simulink library "libMdl_Imm"  (R2019b)
settings: Solver=VariableStepAuto  StartTime=0.0  StopTime=10.0  RelTol=1e-3
undefined symbols (not defined in the file or in its folder): imm_measurement_fcns, imm_mu_sample_time, imm_residuum_fcns, imm_sample_time, imm_state_transition_fcns, mu_0, P_0_imm, Pi, x_0_imm
settings Model: Creator=hwinter  LastModifiedBy=Hanno
settings DataIOCC: ReturnWorkspaceOutputs=off
settings DebuggingCC: ArithmeticOperatorsInVariantConditions=warning
settings SFSimCC: SimUseLocalCustomCode=off  CustomCodeUndefinedFunction=UseInterfaceOnly
settings RTWCC: RTWUseLocalCustomCode=off

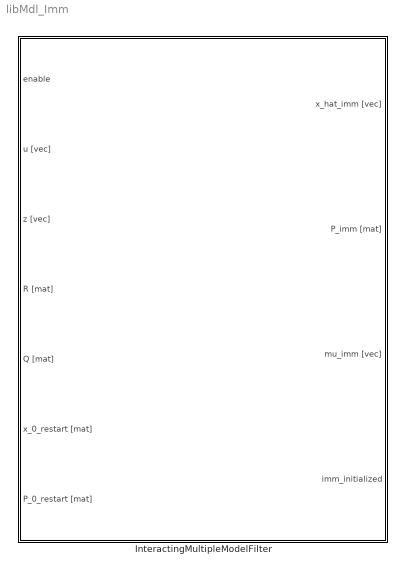
== system libMdl_Imm ==
  InteractingMultipleModelFilter : Subsystem  SystemSampleTime=mv_sample_time  mask(Interacting Multiple Model Filter){mv_sample_time=imm_sample_time, mv_mu_sample_time=imm_mu_sample_time, mv_x_0=x_0_imm, mv_P_0=P_0_imm, mv_pi=Pi, mv_mu_0=mu_0, mv_state_transition_functions=imm_state_transition_fcns, mv_measurement_functions=imm_measurement_fcns, mv_residuum_functions=imm_residuum_fcns}
      mask prompts: mv_sample_time "Sample Time:"; mv_mu_sample_time "Model Likelihood Sample Time:"; mv_x_0 "Initial State:"; mv_P_0 "Initial Covariance:"; mv_pi "Pi:"; mv_mu_0 "mu_0:"; mv_state_transition_functions "State Transition Functions:"; mv_measurement_functions "Measurement Functions:"; mv_residuum_functions "Residuum Functions:"
      mask help:
      | Sample Time:
      | Sample time of the block in seconds
      |
      | Initial State:
      | Initial state in correspondens to the state transition functions
      |
      | Initial Covariance:
      | Initial covariance matrix corresponding to the initial state, defined previously
      |
      | Pi:
      | Model Transition probability matrix
      |
      | mu_0:
      | Initial model probabilities
      |
      | State Transition Functions:
      | Names of the state transition functions, which have to be defined somewhere in the Matlab workspace
      | (example: {stateTransitionFcn1,stateTransitionFcn2})
      |
      | Measurement Functions:
      | Names of the measurement functions, which have to be defined somewhere in the Matlab workspace
      | (example: {measurementFcn1,measurementFcn2})
      |
      | Residuum Functions:
      | Optional functions to calculate measurement innovation (e.g. if angles are included). Leave '[]' if not needed.
      | (example: {residuumFcn1,residuumFcnFcn2})
      mask init:
      | % [mv_state_transition_functions,mv_measurement_functions] = simFcn_Imm_MaskInit(mv_state_transition_functions,mv_measurement_functions);
      | [mv_state_transition_functions,mv_measurement_functions,mv_residuum_functions] = simFcn_Imm_MaskInit(mv_state_transition_functions,mv_measurement_functions,mv_residuum_functions);
      mask Display:
      | str1 = sprintf('\\color{black}{\\bfIMM Filter}\n\n');
      | str2 = sprintf('Sample Time: %0.2f\n',mv_sample_time);
      | str3 = sprintf('Model Likelihood Sample Time: %0.2f\n\n',mv_mu_sample_time);
      | if length(mv_x_0) <= 3
      |     str4 = sprintf('x_0: %s\n',mat2str(mv_x_0,5));
      | else
      |     str4 = sprintf('x_0: [...]\n');
      | end % if
      | if length(mv_P_0) == 1
      |     str5 = sprintf('P_0: %0.2f\n\n',mv_P_0);
      | else
      |     str5 = sprintf('P_0: [...]\n\n');
      | end % if
      | str6 = sprintf('\\Pi: [...]\n');
      | if length(mv_mu_0) <= 3
      |     str7 = sprintf('\\mu_0: %s\n\n',mat2str(mv_mu_0,5));
      | else
      |     str7 = sprintf('\\mu_0: [...]\n\n');
      | end % if
      | str8 = sprintf('State Transition Functions: [...]\n');
      | str9 = sprintf('Measurement Functions: [...]\n');
      | if isempty(mv_residuum_functions)
      |     str10 = '';
      | else
      |     str10 = sprintf('Residuum Functions: [...]');
      | end % if
      | 
      | str = [str1,str2,str3,str4,str5,str6,str7,str8,str9,str10];
      | 
      | text( 0.5,0.5, ...
      |       str, ...
      |       'horizontalAlignment', 'center', ...
      |       'texmode','on' ...
      |     )

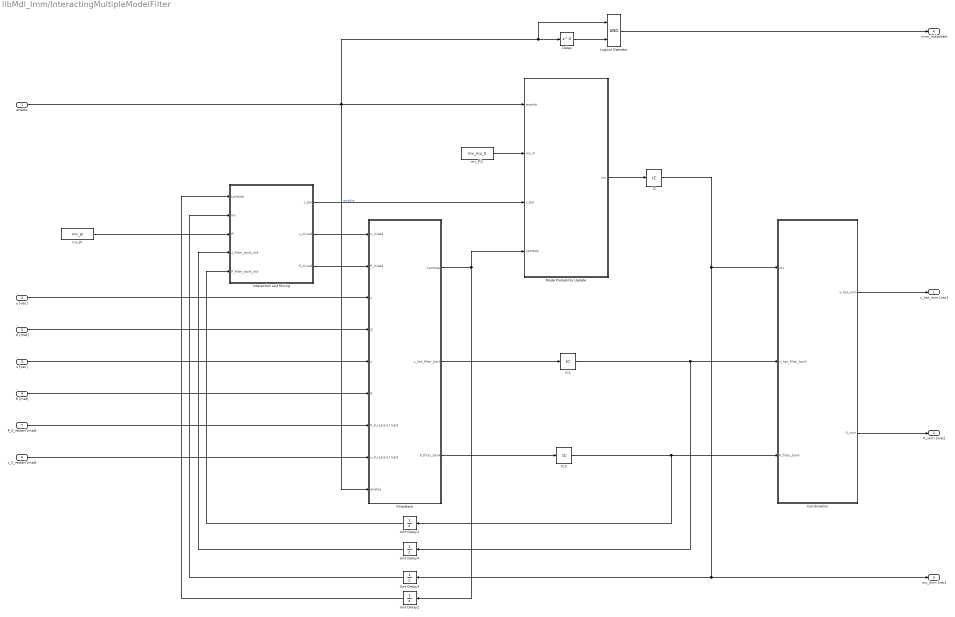
== system libMdl_Imm/InteractingMultipleModelFilter ==
  enable : Inport  SampleTime=mv_sample_time
  u [vec] : Inport  Port=2  SampleTime=mv_sample_time
  z [vec] : Inport  Port=3  SampleTime=mv_sample_time
  R [mat] : Inport  Port=4  SampleTime=mv_sample_time
  Q [mat] : Inport  Port=5  SampleTime=mv_sample_time
  x_0_restart [mat] : Inport  Port=6  SampleTime=mv_sample_time
  P_0_restart [mat] : Inport  Port=7  SampleTime=mv_sample_time
  Combination : Subsystem
  Delay : Delay
  FilterBank : Subsystem  SystemSampleTime=mv_sample_time
  IC : InitialCondition  Value=mv_mu_0
  IC1 : InitialCondition  Value=mv_x_0
  IC2 : InitialCondition  Value=mv_P_0
  Interaction and Mixing : Subsystem  TreatAsAtomicUnit=on
  Logical Operator : Logic  AllPortsSameDT=off  OutDataTypeStr=boolean
  Mode Probability Update : Subsystem
  Unit Delay1 : UnitDelay  InitialCondition=mv_P_0  SampleTime=-1  HasFrameUpgradeWarning=on
  Unit Delay2 : UnitDelay  InitialCondition=NaN(size(mv_mu_0))  SampleTime=-1  HasFrameUpgradeWarning=on
  Unit Delay3 : UnitDelay  InitialCondition=mv_mu_0  SampleTime=-1  HasFrameUpgradeWarning=on
  Unit Delay4 : UnitDelay  InitialCondition=mv_x_0  SampleTime=-1  HasFrameUpgradeWarning=on
  mv_Pi : Constant  Value=mv_pi
  mv_Pi1 : Constant  Value=mv_mu_0
  x_hat_imm [vec] : Outport  VectorParamsAs1DForOutWhenUnconnected=off
  P_imm [mat] : Outport  Port=2  VectorParamsAs1DForOutWhenUnconnected=off
  mu_imm [vec] : Outport  Port=3  VectorParamsAs1DForOutWhenUnconnected=off
  imm_initialized : Outport  Port=4  VectorParamsAs1DForOutWhenUnconnected=off
  wires:
  Logical Operator/1 -> imm_initialized/1
  Delay/1 -> Logical Operator/2
  P_0_restart [mat]/1 -> FilterBank/7(P_0_restart [mat])
  x_0_restart [mat]/1 -> FilterBank/8(x_0_restart [mat])
  enable/1 -> FilterBank/9(enable), Mode Probability Update/1(enable), Delay/1, Logical Operator/1  "enable"
  Unit Delay4/1 -> Interaction and Mixing/4(x_filter_bank_old)
  Unit Delay2/1 -> Interaction and Mixing/1(Lambda)
  mv_Pi1/1 -> Mode Probability Update/2(mu_0)
  IC2/1 -> Combination/3(P_filter_bank), Unit Delay1/1
  IC1/1 -> Combination/2(x_hat_filter_bank), Unit Delay4/1
  Mode Probability Update/1(mu) -> IC/1
  IC/1 -> Combination/1(mu), mu_imm [vec]/1, Unit Delay3/1
  Unit Delay3/1 -> Interaction and Mixing/2(mu)
  Unit Delay1/1 -> Interaction and Mixing/5(P_filter_bank_old)
  FilterBank/2(x_hat_filter_bank) -> IC1/1
  FilterBank/3(P_filter_bank) -> IC2/1
  Combination/1(x_hat_imm) -> x_hat_imm [vec]/1
  Combination/2(P_imm) -> P_imm [mat]/1
  Interaction and Mixing/1(c_bar) -> Mode Probability Update/3(c_bar)
  FilterBank/1(Lambda) -> Unit Delay2/1, Mode Probability Update/4(Lambda)
  mv_Pi/1 -> Interaction and Mixing/3(Pi)
  Interaction and Mixing/3(P_mixed) -> FilterBank/2(P_mixed)
  Interaction and Mixing/2(x_mixed) -> FilterBank/1(x_mixed)
  Q [mat]/1 -> FilterBank/4(Q)
  R [mat]/1 -> FilterBank/6(R)
  z [vec]/1 -> FilterBank/5(z)
  u [vec]/1 -> FilterBank/3(u)

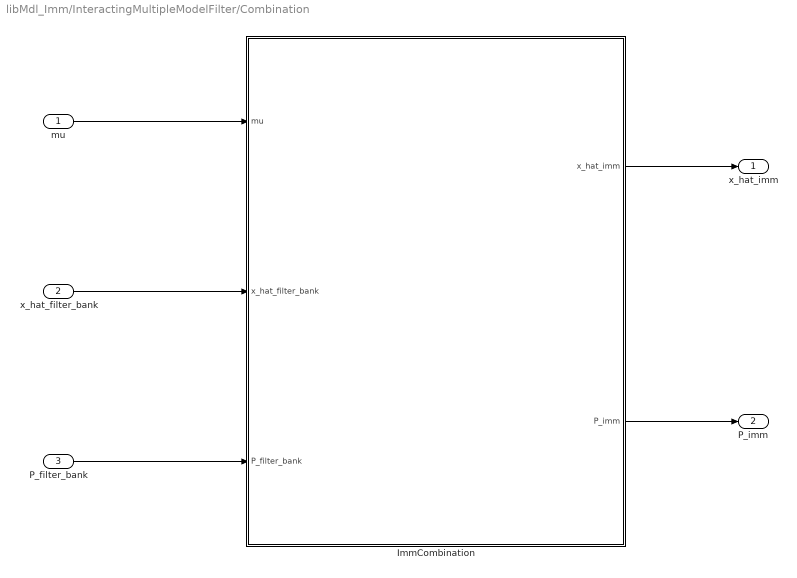
== system libMdl_Imm/InteractingMultipleModelFilter/Combination ==
  mu : Inport
  x_hat_filter_bank : Inport  Port=2
  P_filter_bank : Inport  Port=3
  ImmCombination : MATLAB Function  TreatAsAtomicUnit=on
  x_hat_imm : Outport  VectorParamsAs1DForOutWhenUnconnected=off
  P_imm : Outport  Port=2  VectorParamsAs1DForOutWhenUnconnected=off
  wires:
  ImmCombination/1(x_hat_imm) -> x_hat_imm/1
  ImmCombination/2(P_imm) -> P_imm/1
  mu/1 -> ImmCombination/1(mu)
  x_hat_filter_bank/1 -> ImmCombination/2(x_hat_filter_bank)
  P_filter_bank/1 -> ImmCombination/3(P_filter_bank)

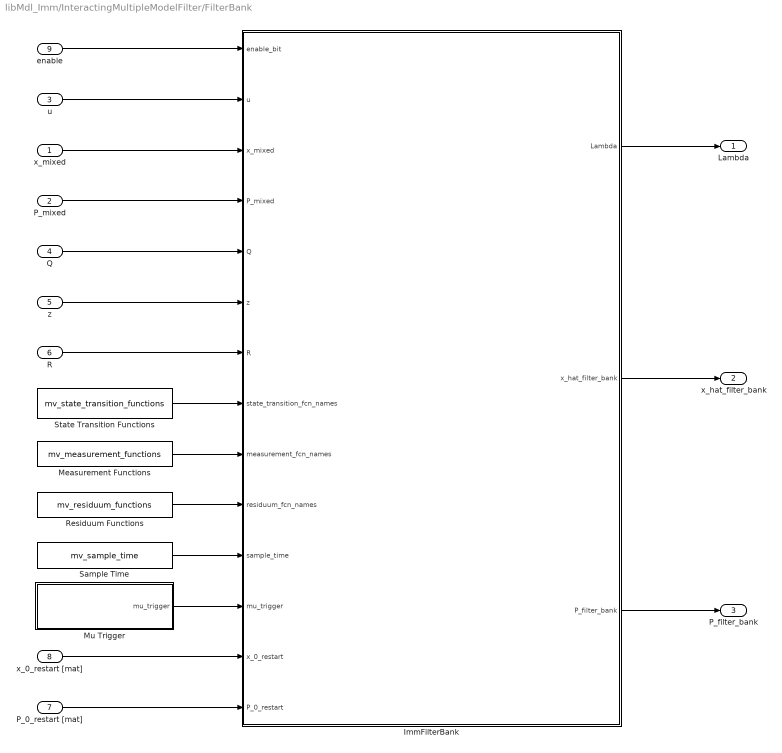
== system libMdl_Imm/InteractingMultipleModelFilter/FilterBank ==
  x_mixed : Inport
  P_mixed : Inport  Port=2
  u : Inport  Port=3
  Q : Inport  Port=4
  z : Inport  Port=5
  R : Inport  Port=6
  P_0_restart [mat] : Inport  Port=7
  x_0_restart [mat] : Inport  Port=8
  enable : Inport  Port=9
  ImmFilterBank : MATLAB Function  TreatAsAtomicUnit=on  SystemSampleTime=mv_sample_time
  Measurement Functions : Constant  Value=mv_measurement_functions
  Mu Trigger : Subsystem
  Residuum Functions : Constant  Value=mv_residuum_functions
  Sample Time : Constant  Value=mv_sample_time
  State Transition Functions : Constant  Value=mv_state_transition_functions
  Lambda : Outport  VectorParamsAs1DForOutWhenUnconnected=off
  x_hat_filter_bank : Outport  Port=2  VectorParamsAs1DForOutWhenUnconnected=off
  P_filter_bank : Outport  Port=3  VectorParamsAs1DForOutWhenUnconnected=off
  wires:
  P_0_restart [mat]/1 -> ImmFilterBank/14(P_0_restart)
  x_0_restart [mat]/1 -> ImmFilterBank/13(x_0_restart)
  enable/1 -> ImmFilterBank/1(enable_bit)
  Mu Trigger/1(mu_trigger) -> ImmFilterBank/12(mu_trigger)
  Residuum Functions/1 -> ImmFilterBank/10(residuum_fcn_names)
  Sample Time/1 -> ImmFilterBank/11(sample_time)
  Measurement Functions/1 -> ImmFilterBank/9(measurement_fcn_names)
  State Transition Functions/1 -> ImmFilterBank/8(state_transition_fcn_names)
  R/1 -> ImmFilterBank/7(R)
  z/1 -> ImmFilterBank/6(z)
  P_mixed/1 -> ImmFilterBank/4(P_mixed)
  Q/1 -> ImmFilterBank/5(Q)
  x_mixed/1 -> ImmFilterBank/3(x_mixed)
  u/1 -> ImmFilterBank/2(u)
  ImmFilterBank/3(P_filter_bank) -> P_filter_bank/1
  ImmFilterBank/2(x_hat_filter_bank) -> x_hat_filter_bank/1
  ImmFilterBank/1(Lambda) -> Lambda/1

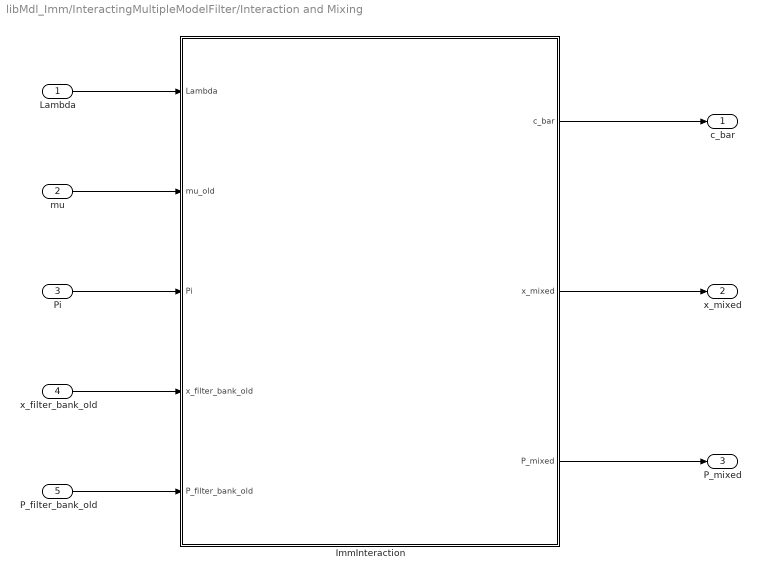
== system libMdl_Imm/InteractingMultipleModelFilter/Interaction and Mixing ==
  Lambda : Inport
  mu : Inport  Port=2
  Pi : Inport  Port=3
  x_filter_bank_old : Inport  Port=4
  P_filter_bank_old : Inport  Port=5
  ImmInteraction : MATLAB Function
  c_bar : Outport  VectorParamsAs1DForOutWhenUnconnected=off
  x_mixed : Outport  Port=2  VectorParamsAs1DForOutWhenUnconnected=off
  P_mixed : Outport  Port=3  VectorParamsAs1DForOutWhenUnconnected=off
  wires:
  Lambda/1 -> ImmInteraction/1(Lambda)
  mu/1 -> ImmInteraction/2(mu_old)
  ImmInteraction/1(c_bar) -> c_bar/1
  Pi/1 -> ImmInteraction/3(Pi)
  x_filter_bank_old/1 -> ImmInteraction/4(x_filter_bank_old)
  P_filter_bank_old/1 -> ImmInteraction/5(P_filter_bank_old)
  ImmInteraction/3(P_mixed) -> P_mixed/1
  ImmInteraction/2(x_mixed) -> x_mixed/1

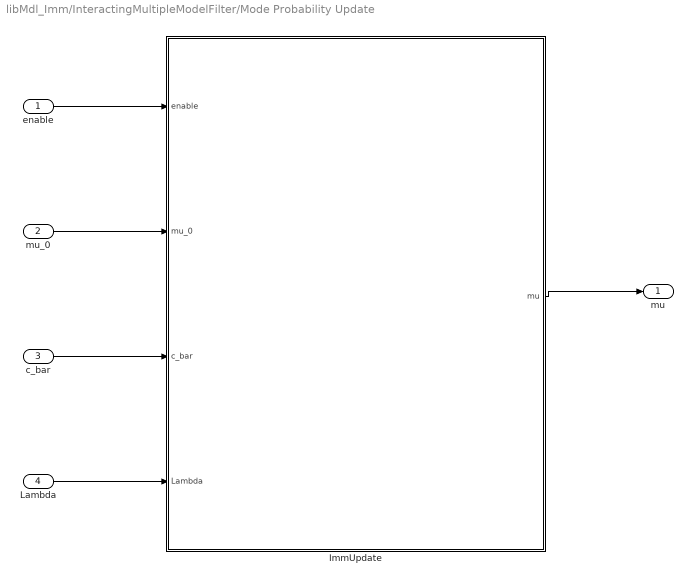
== system libMdl_Imm/InteractingMultipleModelFilter/Mode Probability Update ==
  enable : Inport
  mu_0 : Inport  Port=2
  c_bar : Inport  Port=3
  Lambda : Inport  Port=4
  ImmUpdate : MATLAB Function
  mu : Outport  VectorParamsAs1DForOutWhenUnconnected=off
  wires:
  enable/1 -> ImmUpdate/1(enable)
  mu_0/1 -> ImmUpdate/2(mu_0)
  ImmUpdate/1(mu) -> mu/1
  Lambda/1 -> ImmUpdate/4(Lambda)
  c_bar/1 -> ImmUpdate/3(c_bar)

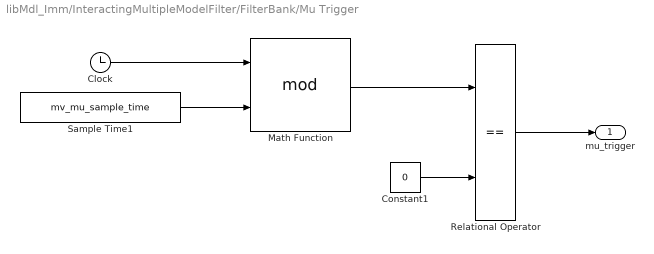
== system libMdl_Imm/InteractingMultipleModelFilter/FilterBank/Mu Trigger ==
  Clock : Clock
  Constant1 : Constant  Value=0
  Math Function : Math  Operator=mod  SignedPower=off  SaturateOnIntegerOverflow=on
  Relational Operator : RelationalOperator  Operator===  OutDataTypeStr=boolean  RndMeth=Simplest
  Sample Time1 : Constant  Value=mv_mu_sample_time
  mu_trigger : Outport
  wires:
  Relational Operator/1 -> mu_trigger/1
  Clock/1 -> Math Function/1
  Constant1/1 -> Relational Operator/2
  Sample Time1/1 -> Math Function/2
  Math Function/1 -> Relational Operator/1

== matlab function libMdl_Imm/InteractingMultipleModelFilter/Combination/ImmCombination ==
  data: mu input; x_hat_imm output; x_hat_filter_bank input; P_filter_bank input; P_imm output
function [x_hat_imm,P_imm] = simFcn_ImmCombination(mu,x_hat_filter_bank,P_filter_bank)
%
% See:  
%   Y. Bar-Shalom et al., 'Estimation with applications to tracking and navigation: theory algorithms and software', 2001, Section 11.6.6, P.455ff.
%

% Init ____________________________________________________________________

% Calculations ____________________________________________________________

% x_k_imm
x_hat_imm = zeros(size(x_hat_filter_bank,1),1);
for j = 1:length(mu)
    x_hat_imm = x_hat_imm + mu(j)*x_hat_filter_bank(:,j);
end % for j

% P_k_imm
P_imm = zeros(size(P_filter_bank,1),size(P_filter_bank,2));
for j = 1:length(mu)
    P_imm = P_imm + mu(j)*(P_filter_bank(:,:,j)+(x_hat_filter_bank(:,j)-x_hat_imm)*(x_hat_filter_bank(:,j)-x_hat_imm)');
end % for j

end % end

== matlab function libMdl_Imm/InteractingMultipleModelFilter/FilterBank/ImmFilterBank ==
  data: enable_bit input; u input; x_mixed input; P_mixed input; Q input; z input; R input; Lambda output; state_transition_fcn_names input; measurement_fcn_names input; residuum_fcn_names input; sample_time input; x_hat_filter_bank output; P_filter_bank output; mu_trigger input; x_0_restart input; P_0_restart input
function [Lambda,x_hat_filter_bank,P_filter_bank] = simFcn_ImmFilterBank(enable_bit,u,x_mixed,P_mixed,Q,z,R,state_transition_fcn_names,measurement_fcn_names,residuum_fcn_names,sample_time,mu_trigger,x_0_restart,P_0_restart)
%
% See:  
%   Y. Bar-Shalom et al., 'Estimation with applications to tracking and navigation: theory algorithms and software', 2001, Section 11.6.6, P.455ff.
%

coder.extrinsic('calcDiscreteKalmanFilter','invChol_mex','bdroot','get_param');

x_hat_filter_bank = coder.nullcopy(zeros([size(x_mixed,1) size(state_transition_fcn_names,1)]));
P_filter_bank = coder.nullcopy(zeros([size(x_mixed,1) size(x_mixed,1) size(state_transition_fcn_names,1)]));
Lambda = coder.nullcopy(zeros([size(state_transition_fcn_names,1) 1]));

persistent mem_var_first_run

% Init ____________________________________________________________________

if isempty(mem_var_first_run)    
    mem_var_first_run = false;
    
    x_hat_filter_bank = NaN(size(x_mixed));
    P_filter_bank = NaN(size(P_mixed));
    Lambda = NaN(size(Lambda,1),1);
    
    return
end % if

if ~enable_bit
    x_hat_filter_bank = x_0_restart;
    P_filter_bank = P_0_restart;
    Lambda = NaN(size(Lambda,1),1);
    
    return
end % if



% Calculations ____________________________________________________________
for i = 1:size(state_transition_fcn_names,1)
    
    % extract string from input and remove padded spaces
    state_transition_fcn_string_i = char(state_transition_fcn_names(i,state_transition_fcn_names(i,:)~=32));
    measurement_fcn_string_i = char(measurement_fcn_names(i,measurement_fcn_names(i,:)~=32));
    residuum_fcn_string_i = char(residuum_fcn_names(i,residuum_fcn_names(i,:)~=32));
       
    % filtering
    [x_hat_filter_bank(:,i),P_filter_bank(:,:,i),nu,S] = calcDiscreteKalmanFilter(u,z,Q(:,:,i),R,x_mixed(:,i),P_mixed(:,:,i),state_transition_fcn_string_i,measurement_fcn_string_i,sample_time,residuum_fcn_string_i);
        
    valid_measurement_selector = ( (z~=0) & (diag(R)~=0) );
        
    if any(valid_measurement_selector) && mu_trigger      
        % Lambda(i) = 1/sqrt(det(2*pi*S))*exp(-1/2*nu'*S^-1*nu);
        Lambda(i) = 1/sqrt(det(2*pi*S))*exp( -1/2*nu' * invChol_mex(S) * nu );
        
        if all(Lambda == 0)
            Lambda = nan(size(Lambda));
            
            sim_time = get_param(bdroot,'SimulationTime');            
            disp(['Time: ',sprintf('%.2f',sim_time),' -- IMM Filter: All model likelihoods are equal to zero. Skipped likelihood update!'])
        end % if
    else
        Lambda(i) = NaN;
    end % if   
    
end % for

end % function

== matlab function libMdl_Imm/InteractingMultipleModelFilter/Interaction and Mixing/ImmInteraction ==
  data: Lambda input; c_bar output; mu_old input; Pi input; x_mixed output; x_filter_bank_old input; P_filter_bank_old input; P_mixed output
function [c_bar,x_mixed,P_mixed] = simFcn_ImmInteraction(Lambda,mu_old,Pi,x_filter_bank_old,P_filter_bank_old)
%
% See:  
%   Y. Bar-Shalom et al., 'Estimation with applications to tracking and navigation: theory algorithms and software', 2001, Section 11.6.6, P.455ff.
%


% Checks and Initialization _______________________________________________

% Check Pi
for i = 1:size(Pi,1)
    p_i = sum(Pi(i,:));    
    if p_i ~= 1
        error('''Pi'' is not choosen correctly!');
    end % if
end % for i

% Calculations ____________________________________________________________

switch ~any(isnan(Lambda))
    case 1
       
        c_bar = zeros(size(mu_old));
        mu_mixed_old = zeros(length(mu_old));
        x_mixed = zeros(size(x_filter_bank_old));
        P_mixed = zeros(size(P_filter_bank_old));

        % normalization constant c_bar
        for j = 1:length(c_bar)
            for i = 1:length(c_bar)
                c_bar(j) = c_bar(j) + Pi(i,j) *  mu_old(i);
            end % for i
        end % for j

        % mu_mixing_k_old
        for i = 1:length(c_bar)
            for j = 1:length(c_bar)
                mu_mixed_old(i,j) = (Pi(i,j) * mu_old(i)) / c_bar(j);
            end % for j
        end % for i

        % x_mixed
        for j = 1:length(c_bar)
            for i = 1:length(c_bar)
                x_mixed(:,j) = x_mixed(:,j) + x_filter_bank_old(:,i)*mu_mixed_old(i,j);
            end % for i
        end % for r

        % P_mixed
        for j = 1:length(c_bar)
            for i = 1:length(c_bar)
                P_mixed(:,:,j) = P_mixed(:,:,j) + mu_mixed_old(i,j)*(P_filter_bank_old(:,:,i) + (x_filter_bank_old(:,i)-x_mixed(:,j))*(x_filter_bank_old(:,i)-x_mixed(:,j))');
            end % for i
        end % for r
        
    otherwise
        
        c_bar = zeros(size(mu_old));        
        for j = 1:length(c_bar)
            for i = 1:length(c_bar)
                c_bar(j) = c_bar(j) + Pi(i,j) *  mu_old(i);
            end % for i
        end % for j
        
        x_mixed = x_filter_bank_old;
        P_mixed = P_filter_bank_old;
        
end % switch



end % end function

== matlab function libMdl_Imm/InteractingMultipleModelFilter/Mode Probability Update/ImmUpdate ==
  data: enable input; mu_0 input; c_bar input; mu output; Lambda input
function mu = simFcn_ImmUpdate(enable,mu_0,c_bar,Lambda)
%
% See:  
%   Y. Bar-Shalom et al., 'Estimation with applications to tracking and navigation: theory algorithms and software', 2001, Section 11.6.6, P.455ff.
%

% Init ____________________________________________________________________

persistent mem_var_mu

if isempty(mem_var_mu)
    mem_var_mu = mu_0;
end % if

if ~enable
%     mem_var_mu = mu_0;
%     mu = mu_0;
    mu = mem_var_mu;
    return
end % if

% Calculations ____________________________________________________________

switch ~any(isnan(Lambda))
    case 1
       
        c = 0;
        for i = 1:length(c_bar)
            c = c + c_bar(i) * Lambda(i);
        end % for i

        mu = zeros(size(c_bar));
        for j = 1:length(c_bar)
            mu(j) = (Lambda(j) * c_bar(j)) / c;
        end % for i
        
        mem_var_mu = mu;
        
    otherwise
        
        mu = mem_var_mu;
        
end % switch

end % end function
